simulink library "COR_lib"  (Simulink 7.4)
settings: Solver=FixedStepDiscrete  StartTime=0.0  StopTime=Inf  FixedStep=0.01  RelTol=1e-3
values from neighbouring files (symbols this model uses):
  CORc_fac_CellRDcse_fault = mpt.Parameter    [COR_CAL.m]
  CORc_fac_CellRDcse_warn = mpt.Parameter    [COR_CAL.m]
  CORc_i_ChaEndCur = mpt.Parameter    [COR_CAL.m]
  CORc_i_SOCCrectCurThrld = mpt.Parameter    [COR_CAL.m]
  CORc_pct_DeltSoe_max = mpt.Parameter    [COR_CAL.m]
  CORc_pct_DeltSoe_min = mpt.Parameter    [COR_CAL.m]
  CORc_pct_SOCModValue = mpt.Parameter    [COR_CAL.m]
  CORc_v_CellVoltMax = mpt.Parameter    [COR_CAL.m]
undefined symbols (not defined in the file or in its folder): BATd_iflt_CellCDcse_fault, BATd_pct_CellCVariMax, BATd_pct_CellCVariMin, BATd_v_CellUpperVolt, BATd_v_PackVoltMin, BATm_c_CellChaC_AH, BATm_c_CellDchC_AH, BATm_e_CellSoe, BATm_e_ChaCellSoe, BATm_e_DchCellSoe, BATm_i_PerChaCur, BATm_i_PerDchCur, BATm_i_PulChaCur_limit, BATm_i_PulDchCur_limit, BATm_i_PulDchVolt_limit, BATm_pct_CellCDcseRatio, BATm_pct_CellCycle, BATm_pct_CellSoc, BATm_pct_ChaCellSoc, BATm_pct_DchCellSoc, BATm_pct_SOCofOCVPct, BATm_pct_SohRatio, BATm_r_ChaDcIR, BATm_r_DchDcIR, BATm_v_CellOCV, BATx_pct_CellSocRatio, BATx_pct_PackSoh, BATx_t_CellChaTemp, BATx_t_CellDchTemp, BATx_tm_OfflineTime, BATy_i_CellChaCur, BATy_i_CellDchCur, BATz_v_CellChaVolt, BATz_v_DchCellVolt, BATz_v_DchCellVoltForSoe, BCU_FastCharge_St, BCU_SlowCharge_St, BMS_Const_TickTm_s, BMU_Run_St, FCM_Charging_St, PACK_Const_CellNumOfMdl, PACK_Const_CellNumOfPack, PACK_Const_CycCnt, PACK_Const_MdlNumOfPack, PACK_Const_ParaCellNumOfMdl, PACK_Const_TempSnrNumOfMdl, SCM_Charging_St
libraries: Defined_Functionality x17
(part 2 of 2)

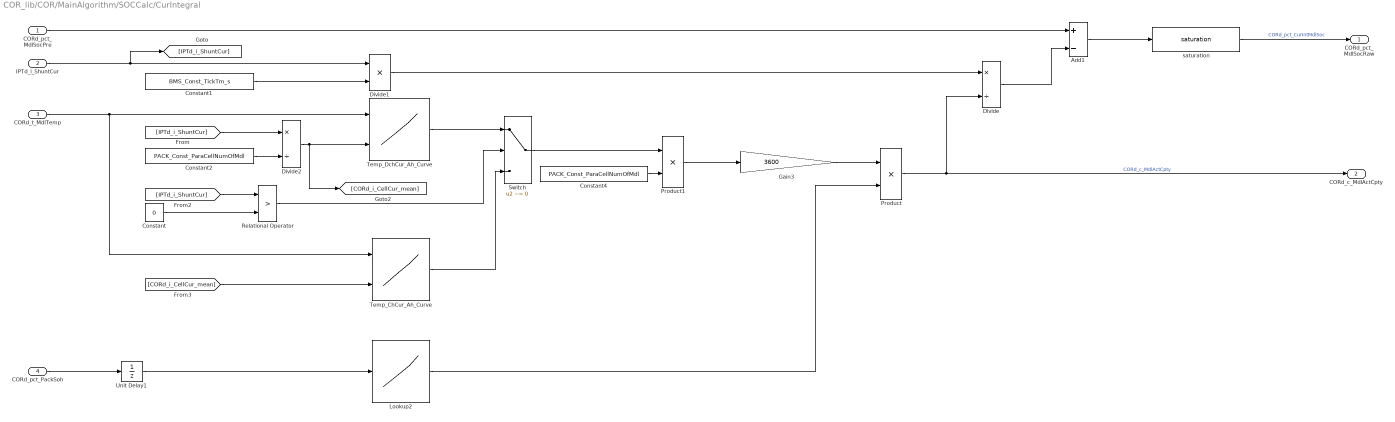
== system COR_lib/COR/MainAlgorithm/SOCCalc/CurIntegral ==
  CORd_pct_MdlSocPre : Inport
  IPTd_i_ShuntCur : Inport  Port=2
  CORd_t_MdlTemp : Inport  Port=3
  CORd_pct_PackSoh : Inport  Port=4  DataType=single  OutDataTypeStr=single
  Add1 : Sum  Inputs=+-
  Constant : Constant  Value=0  OutDataTypeMode=single  OutDataType=fixdt(1, 16)  OutScaling=2^0  OutDataTypeStr=single
  Constant1 : Constant  Value=BMS_Const_TickTm_s  OutDataTypeMode=single  OutDataType=fixdt(1, 16)  OutScaling=2^0  OutDataTypeStr=single
  Constant2 : Constant  Value=PACK_Const_ParaCellNumOfMdl  OutDataTypeMode=single  OutDataType=fixdt(1, 16)  OutScaling=2^0  OutDataTypeStr=single
  Constant4 : Constant  Value=PACK_Const_ParaCellNumOfMdl  OutDataTypeMode=single  OutDataType=fixdt(1, 16)  OutScaling=2^0  OutDataTypeStr=single
  Divide : Product  Inputs=*/
  Divide1 : Product  Inputs=**
  Divide2 : Product  Inputs=*/
  Gain3 : Gain  Gain=3600
  Lookup2 : Lookup  InputValues=BATx_pct_PackSoh  Table=BATm_pct_CellCDcseRatio  LookUpMeth=Interpolation-Use End Values  OutDataType=fixdt(1, 16)  OutScaling=2^0
  Product : Product  OutDataType=fixdt(1, 16)  OutScaling=2^0  RndMeth=Zero
  Product1 : Product  OutDataType=fixdt(1, 16)  OutScaling=2^0  RndMeth=Zero
  Relational Operator : RelationalOperator  Operator=>  LogicOutDataTypeMode=boolean  LogicDataType=fixdt(0, 8)  OutDataTypeStr=boolean
  Switch : Switch  Criteria=u2 ~= 0  OutDataType=fixdt(1, 16)  OutScaling=2^0
  Temp_ChCur_Ah_Curve : Lookup2D  RowIndex=BATx_t_CellChaTemp  ColumnIndex=BATy_i_CellChaCur  Table=BATm_c_CellChaC_AH  LookUpMeth=Interpolation-Use End Values  OutDataType=fixdt(1, 16)  OutScaling=2^0
  Temp_DchCur_Ah_Curve : Lookup2D  RowIndex=BATx_t_CellDchTemp  ColumnIndex=BATy_i_CellDchCur  Table=BATm_c_CellDchC_AH  LookUpMeth=Interpolation-Use End Values  OutDataType=fixdt(1, 16)  OutScaling=2^0
  Unit Delay1 : UnitDelay  SampleTime=-1
  saturation : Defined_Functionality/saturation  SystemSampleTime=-1  upper_limit=1  lower_limit=0
      settings: AttributesFormatString=[UPPER_LIMIT=%<upper_limit>]\n[LOWER_LIMIT=%<lower_limit>]
  CORd_pct_MdlSocRaw : Outport
  CORd_c_MdlActCpty : Outport  Port=2
  wires:
  saturation/1 -> CORd_pct_MdlSocRaw/1  "CORd_pct_CurIntMdlSoc"
  [CORd_i_CellCur_mean] -> Temp_ChCur_Ah_Curve/2
  Divide1/1 -> Divide/1
  Divide/1 -> Add1/2
  Add1/1 -> saturation/1
  IPTd_i_ShuntCur/1 -> [IPTd_i_ShuntCur], Divide1/1
  CORd_t_MdlTemp/1 -> Temp_DchCur_Ah_Curve/1, Temp_ChCur_Ah_Curve/1
  CORd_pct_MdlSocPre/1 -> Add1/1
  [IPTd_i_ShuntCur] -> Relational Operator/1
  Constant/1 -> Relational Operator/2
  Relational Operator/1 -> Switch/2
  Temp_DchCur_Ah_Curve/1 -> Switch/1
  Temp_ChCur_Ah_Curve/1 -> Switch/3
  Switch/1 -> Product1/1
  Constant1/1 -> Divide1/2
  Product/1 -> CORd_c_MdlActCpty/1, Divide/2  "CORd_c_MdlActCpty"
  Lookup2/1 -> Product/2
  CORd_pct_PackSoh/1 -> Unit Delay1/1
  Gain3/1 -> Product/1
  Divide2/1 -> [CORd_i_CellCur_mean], Temp_DchCur_Ah_Curve/2
  [IPTd_i_ShuntCur] -> Divide2/1
  Constant2/1 -> Divide2/2
  Constant4/1 -> Product1/2
  Product1/1 -> Gain3/1
  Unit Delay1/1 -> Lookup2/1

== system COR_lib/COR/MainAlgorithm/SOCCalc/EndSOCCalc ==
  CORd_flg_DchEnd : Inport
  Cord_i_ShuntCur_mean : Inport  Port=2
  CORd_t_MdlTemp : Inport  Port=3
  CORd_v_CellVoltOfMdl_mean : Inport  Port=4
  ChaEndSocCalc : Subsystem
  DchEndSocCalc : Subsystem
  Logical Operator4 : Logic  Operator=NOT  AllPortsSameDT=off  OutDataTypeMode=boolean  LogicDataType=fixdt(0, 8)  OutDataTypeStr=boolean
  Switch : Switch  Criteria=u2 ~= 0  OutDataType=fixdt(1, 16)  OutScaling=2^0
  CORd_pct_EndMdlSoc : Outport
  wires:
  [CORd_t_MdlTemp] -> ChaEndSocCalc/3(CORd_t_MdlTemp)
  [CORd_v_CellVoltOfMdl_mean] -> ChaEndSocCalc/2(CORd_v_CellVoltOfMdl_mean)
  [Cord_i_ShuntCur_mean] -> ChaEndSocCalc/1(Cord_i_ShuntCur_mean)
  Cord_i_ShuntCur_mean/1 -> [Cord_i_ShuntCur_mean], DchEndSocCalc/1(Cord_i_ShuntCur_mean)
  CORd_t_MdlTemp/1 -> DchEndSocCalc/3(CORd_t_MdlTemp), [CORd_t_MdlTemp]
  CORd_v_CellVoltOfMdl_mean/1 -> DchEndSocCalc/2(CORd_v_CellVoltOfMdl_mean), [CORd_v_CellVoltOfMdl_mean]
  DchEndSocCalc/1(CORd_pct_DchEndMdlSoc) -> Switch/1
  Switch/1 -> CORd_pct_EndMdlSoc/1  "CORd_pct_EndMdlSoc"
  [CORd_flg_DchEnd] -> Logical Operator4/1
  Logical Operator4/1 -> ChaEndSocCalc/Enable
  [CORd_flg_DchEnd] -> Switch/2
  CORd_flg_DchEnd/1 -> DchEndSocCalc/Enable, [CORd_flg_DchEnd]
  ChaEndSocCalc/1(CORd_pct_ChEndMdlSoc) -> Switch/3

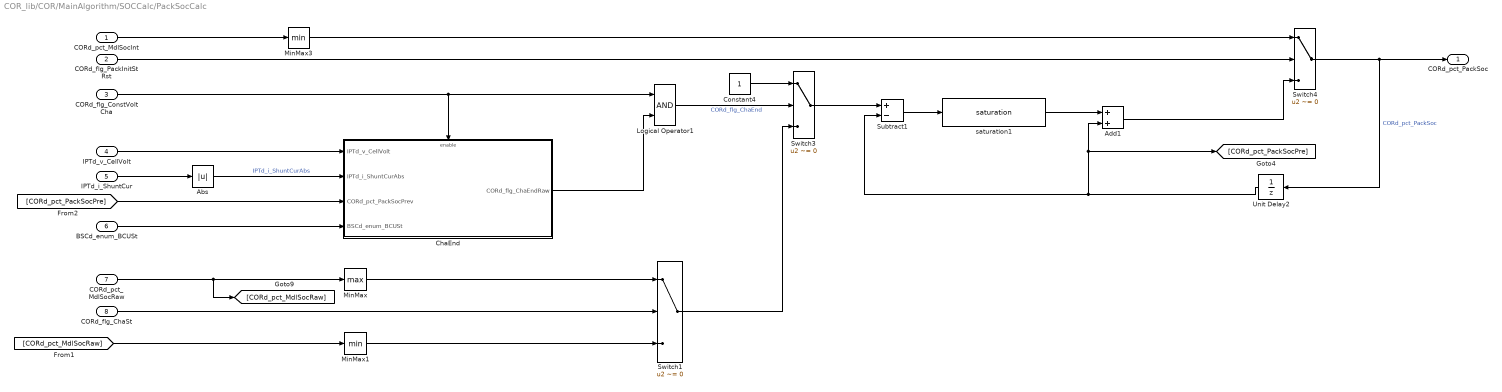
== system COR_lib/COR/MainAlgorithm/SOCCalc/PackSocCalc ==
  CORd_pct_MdlSocInt : Inport
  CORd_flg_PackInitStRst : Inport  Port=2
  CORd_flg_ConstVoltCha : Inport  Port=3
  IPTd_v_CellVolt : Inport  Port=4
  IPTd_i_ShuntCur : Inport  Port=5
  BSCd_enum_BCUSt : Inport  Port=6
  CORd_pct_MdlSocRaw : Inport  Port=7
  CORd_flg_ChaSt : Inport  Port=8
  Abs : Abs  OutDataType=fixdt(1, 16)  OutScaling=2^0
  Add1 : Sum  OutDataType=fixdt(1, 16)  OutScaling=2^-10
  ChaEnd : Subsystem
  Constant4 : Constant  OutDataTypeMode=single  OutDataType=fixdt(1, 16)  OutScaling=2^0  OutDataTypeStr=single
  Logical Operator1 : Logic  AllPortsSameDT=off  OutDataTypeMode=boolean  LogicDataType=fixdt(0, 8)  OutDataTypeStr=boolean
  MinMax : MinMax  Function=max  OutDataType=fixdt(1, 16)  OutScaling=2^0
  MinMax1 : MinMax  OutDataType=fixdt(1, 16)  OutScaling=2^0
  MinMax3 : MinMax  OutDataType=fixdt(1, 16)  OutScaling=2^0
  Subtract1 : Sum  Inputs=+-  OutDataTypeMode=single  OutDataType=fixdt(1, 16)  OutScaling=2^-10  OutDataTypeStr=single
  Switch1 : Switch  Criteria=u2 ~= 0  OutDataType=fixdt(1, 16)  OutScaling=2^0
  Switch3 : Switch  Criteria=u2 ~= 0  OutDataType=fixdt(1, 16)  OutScaling=2^0
  Switch4 : Switch  Criteria=u2 ~= 0  OutDataTypeMode=single  OutDataType=fixdt(1, 16)  OutScaling=2^0  OutDataTypeStr=single
  Unit Delay2 : UnitDelay  SampleTime=-1
  saturation1 : Defined_Functionality/saturation  SystemSampleTime=-1  upper_limit=CORc_pct_DeltSoc_max  lower_limit=CORc_pct_DeltSoc_min
      settings: AttributesFormatString=[UPPER_LIMIT=%<upper_limit>]\n[LOWER_LIMIT=%<lower_limit>]
  CORd_pct_PackSoc : Outport
  wires:
  Switch3/1 -> Subtract1/1
  Unit Delay2/1 -> [CORd_pct_PackSocPre], Add1/2, Subtract1/2
  saturation1/1 -> Add1/1
  MinMax3/1 -> Switch4/1
  Switch4/1 -> CORd_pct_PackSoc/1, Unit Delay2/1  "CORd_pct_PackSoc"
  Subtract1/1 -> saturation1/1
  Add1/1 -> Switch4/3
  CORd_flg_PackInitStRst/1 -> Switch4/2
  CORd_pct_MdlSocInt/1 -> MinMax3/1
  [CORd_pct_MdlSocRaw] -> MinMax1/1
  [CORd_pct_PackSocPre] -> ChaEnd/3(CORd_pct_PackSocPrev)
  Abs/1 -> ChaEnd/2(IPTd_i_ShuntCurAbs)  "IPTd_i_ShuntCurAbs"
  IPTd_i_ShuntCur/1 -> Abs/1
  CORd_flg_ChaSt/1 -> Switch1/2
  Constant4/1 -> Switch3/1
  Logical Operator1/1 -> Switch3/2  "CORd_flg_ChaEnd"
  ChaEnd/1(CORd_flg_ChaEndRaw) -> Logical Operator1/2
  CORd_flg_ConstVoltCha/1 -> ChaEnd/Enable, Logical Operator1/1
  IPTd_v_CellVolt/1 -> ChaEnd/1(IPTd_v_CellVolt)
  Switch1/1 -> Switch3/3
  CORd_pct_MdlSocRaw/1 -> [CORd_pct_MdlSocRaw], MinMax/1
  MinMax1/1 -> Switch1/3
  MinMax/1 -> Switch1/1
  BSCd_enum_BCUSt/1 -> ChaEnd/4(BSCd_enum_BCUSt)

== system COR_lib/COR/MainAlgorithm/SOECalc/EndSoeCalc ==
  CORd_flg_DchEnd : Inport
  CORd_i_ShuntCur_mean : Inport  Port=2
  CORd_v_CellVoltOfMdl_mean : Inport  Port=3
  CORd_t_MdlTemp : Inport  Port=4
  Enable : EnablePort
  ChaEndSoeCal : Subsystem
  DchEndSoeCal : Subsystem
  Logical Operator : Logic  Operator=NOT  AllPortsSameDT=off  OutDataTypeMode=boolean  LogicDataType=fixdt(0, 8)  OutDataTypeStr=boolean
  Switch : Switch  Criteria=u2 ~= 0  OutDataType=fixdt(1, 16)  OutScaling=2^0
  CORd_e_PackSoeRaw2 : Outport
  wires:
  [CORd_t_MdlTemp] -> ChaEndSoeCal/3(CORd_t_MdlTemp)
  [CORd_v_CellVoltOfMdl_mean] -> ChaEndSoeCal/2(CORd_v_CellVoltOfMdl_mean)
  CORd_t_MdlTemp/1 -> [CORd_t_MdlTemp], DchEndSoeCal/3(CORd_t_MdlTemp)
  CORd_v_CellVoltOfMdl_mean/1 -> [CORd_v_CellVoltOfMdl_mean], DchEndSoeCal/2(CORd_v_CellVoltOfMdl_mean)
  [CORd_i_ShuntCur_mean] -> ChaEndSoeCal/1(CORd_i_ShuntCur_mean)
  Switch/1 -> CORd_e_PackSoeRaw2/1  "CORd_e_PackSoeRaw2"
  DchEndSoeCal/1(CORd_e_DchEndCellSoc) -> Switch/1
  ChaEndSoeCal/1(CORd_e_ChaEndCellSoc) -> Switch/3
  CORd_flg_DchEnd/1 -> DchEndSoeCal/Enable, [CORd_flg_DchEnd]
  [CORd_flg_DchEnd] -> Switch/2
  [CORd_flg_DchEnd] -> Logical Operator/1
  Logical Operator/1 -> ChaEndSoeCal/Enable
  CORd_i_ShuntCur_mean/1 -> DchEndSoeCal/1(CORd_i_ShuntCur_mean), [CORd_i_ShuntCur_mean]

== system COR_lib/COR/MainAlgorithm/SOECalc/PackDC-IRCalc ==
  CORd_t_MdlTemp : Inport
  CORd_pct_MdlSoc : Inport  Port=2
  IPTd_i_ShuntCur : Inport  Port=3
  Constant : Constant  OutDataTypeMode=single  OutDataType=fixdt(1, 16)  OutScaling=2^0  OutDataTypeStr=single
  Constant1 : Constant  Value=1000  OutDataTypeMode=single  OutDataType=fixdt(1, 16)  OutScaling=2^0  OutDataTypeStr=single
  Constant2 : Constant  Value=-1  OutDataTypeMode=single  OutDataType=fixdt(1, 16)  OutScaling=2^0  OutDataTypeStr=single
  Constant3 : Constant  Value=0  OutDataTypeMode=single  OutDataType=fixdt(1, 16)  OutScaling=2^0  OutDataTypeStr=single
  Constant4 : Constant  Value=PACK_Const_ParaCellNumOfMdl  OutDataTypeMode=single  OutDataType=fixdt(1, 16)  OutScaling=2^0  OutDataTypeStr=single
  Constant5 : Constant  Value=PACK_Const_CellNumOfMdl  OutDataTypeMode=single  OutDataType=fixdt(1, 16)  OutScaling=2^0  OutDataTypeStr=single
  Divide : Product  Inputs=*/  OutDataType=fixdt(1, 16)  OutScaling=2^-10
  Divide1 : Product  Inputs=*/  OutDataType=fixdt(1, 16)  OutScaling=2^-10
  Product : Product  OutDataType=fixdt(1, 16)  OutScaling=2^0  RndMeth=Zero
  Relational Operator : RelationalOperator  Operator=>  LogicOutDataTypeMode=boolean  LogicDataType=fixdt(0, 8)  OutDataTypeStr=boolean
  Relational Operator1 : RelationalOperator  Operator=<  LogicOutDataTypeMode=boolean  LogicDataType=fixdt(0, 8)  OutDataTypeStr=boolean
  Sum of Elements3 : Sum  Inputs=+  CollapseDim=2  OutDataType=fixdt(1, 16)  OutScaling=2^-10
  Switch : Switch  Criteria=u2 ~= 0  OutDataType=fixdt(1, 16)  OutScaling=2^0
  Switch1 : Switch  Criteria=u2 ~= 0  OutDataType=fixdt(1, 16)  OutScaling=2^0
  T_SOC_ChaDcIR : Lookup2D  RowIndex=BATx_t_CellDchTemp  ColumnIndex=BATy_pct_CellSoc  Table=BATm_r_ChaDcIR  LookUpMeth=Interpolation-Use End Values  OutDataType=fixdt(1, 16)  OutScaling=2^0
  T_SOC_DchDcIR : Lookup2D  RowIndex=BATx_t_CellDchTemp  ColumnIndex=BATy_pct_CellSoc  Table=BATm_r_DchDcIR  LookUpMeth=Interpolation-Use End Values  OutDataTypeMode=single  OutDataType=fixdt(1, 16)  OutScaling=2^0  OutDataTypeStr=single
  CORd_r_CellDCIR : Outport  OutDataType=fixdt(1, 16)  OutScaling=2^0
  CORd_r_PackDCIR : Outport  Port=2  OutDataType=fixdt(1, 16)  OutScaling=2^0
  wires:
  Product/1 -> Sum of Elements3/1
  Divide/1 -> CORd_r_PackDCIR/1  "CORd_r_PackDCIR"
  CORd_t_MdlTemp/1 -> T_SOC_DchDcIR/1, [CORd_t_MdlTemp]
  CORd_pct_MdlSoc/1 -> [CORd_pct_MdlSoc], T_SOC_DchDcIR/2
  IPTd_i_ShuntCur/1 -> Relational Operator/1, Relational Operator1/1
  Constant/1 -> Relational Operator/2
  Relational Operator/1 -> Switch/2
  Switch/1 -> Product/1, CORd_r_CellDCIR/1  "CORd_r_CellDCIR"
  [CORd_pct_MdlSoc] -> T_SOC_ChaDcIR/2
  T_SOC_DchDcIR/1 -> Switch/1
  Constant1/1 -> Divide/2
  [CORd_t_MdlTemp] -> T_SOC_ChaDcIR/1
  T_SOC_ChaDcIR/1 -> Switch1/1
  Constant2/1 -> Relational Operator1/2
  Relational Operator1/1 -> Switch1/2
  Constant3/1 -> Switch1/3
  Switch1/1 -> Switch/3
  Sum of Elements3/1 -> Divide1/1
  Constant4/1 -> Divide1/2
  Divide1/1 -> Divide/1
  Constant5/1 -> Product/2

== system COR_lib/COR/MainAlgorithm/SOECalc/PowInt ==
  note: Note:Not include the energy consumed by the terminals.
  CORd_r_PackDCIR : Inport
  CORd_e_PackSoePre : Inport  Port=2
  CORd_v_CellVoltOfMdl_mean : Inport  Port=3
  IPTd_i_ShuntCur : Inport  Port=4
  Add1 : Sum  Inputs=+-
  Add2 : Sum
  Constant : Constant  Value=3600  OutDataTypeMode=single  OutDataType=fixdt(1, 16)  OutScaling=2^0  OutDataTypeStr=single
  Constant2 : Constant  Value=BMS_Const_TickTm_s  OutDataTypeMode=single  OutDataType=fixdt(1, 16)  OutScaling=2^0  OutDataTypeStr=single
  Constant3 : Constant  Value=3600  OutDataTypeMode=single  OutDataType=fixdt(1, 16)  OutScaling=2^0  OutDataTypeStr=single
  Constant4 : Constant  Value=PACK_Const_CellNumOfMdl  OutDataTypeMode=single  OutDataType=fixdt(1, 16)  OutScaling=2^0  OutDataTypeStr=single
  Divide : Product  Inputs=*/  OutDataType=fixdt(1, 16)  OutScaling=2^-10  OutDataTypeStr=Inherit: Inherit via back propagation
  Divide{1,3..7} (6 alike) : Product  Inputs=**
  Sum of Elements : Sum  Inputs=+  OutDataType=fixdt(1, 16)  OutScaling=2^-10
  CORd_e_PackSoeRaw1 : Outport
  wires:
  Divide5/1 -> Add1/2
  Constant4/1 -> Divide7/2
  Constant3/1 -> Divide6/2
  IPTd_i_ShuntCur/1 -> Divide1/2, Divide4/1, Divide4/2
  Add1/1 -> Divide/1
  CORd_v_CellVoltOfMdl_mean/1 -> Sum of Elements/1
  Divide1/1 -> Add2/1
  CORd_r_PackDCIR/1 -> Divide3/2
  Constant/1 -> Divide/2
  Sum of Elements/1 -> Divide7/1
  Divide4/1 -> Divide3/1
  Divide3/1 -> Add2/2
  Constant2/1 -> Divide5/2
  Divide7/1 -> Divide1/1
  CORd_e_PackSoePre/1 -> Divide6/1
  Divide6/1 -> Add1/1
  Add2/1 -> Divide5/1
  Divide/1 -> CORd_e_PackSoeRaw1/1  "CORd_e_PackSoeRaw1"

== system COR_lib/COR/MainAlgorithm/SOHCalc/SohBaseCycle ==
  CORd_num_RemdCycInt : Inport
  IPTd_i_ShuntCur : Inport  Port=2
  CORd_c_MdlActCpty : Inport  Port=3
  CORd_t_MdlTemp : Inport  Port=4
  Abs : Abs  OutDataType=fixdt(1, 16)  OutScaling=2^0
  Add1 : Sum  Inputs=+-
  Constant : Constant  Value=2  OutDataTypeMode=uint8  OutDataType=fixdt(1, 16)  OutScaling=2^0  OutDataTypeStr=uint8
  Constant1 : Constant  Value=BMS_Const_TickTm_s  OutDataTypeMode=single  OutDataType=fixdt(1, 16)  OutScaling=2^0  OutDataTypeStr=single
  Constant5 : Constant  Value=PACK_Const_CycCnt  OutDataTypeMode=single  OutDataType=fixdt(1, 16)  OutScaling=2^0  OutDataTypeStr=single
  Constant6 : Constant  Value=PACK_Const_MdlNumOfPack  OutDataTypeMode=uint8  OutDataType=fixdt(1, 16)  OutScaling=2^0  OutDataTypeStr=uint8
  Divide : Product  Inputs=*/
  Divide1 : Product  Inputs=**
  Divide2 : Product  Inputs=*/
  Divide3 : Product  Inputs=*/  OutDataType=fixdt(1, 16)  OutScaling=2^-10
  Divide4 : Product  Inputs=*/  OutDataTypeStr=Inherit: Inherit via back propagation
  Divide5 : Product  Inputs=**
  Sum of Elements : Sum  Inputs=+  OutDataType=fixdt(1, 16)  OutScaling=2^-10
  Temp_DchCur_SohRatio : Lookup2D  RowIndex=BATx_t_CellDchTemp  ColumnIndex=BATy_i_CellDchCur  Table=BATm_pct_SohRatio  LookUpMeth=Interpolation-Use End Values  OutDataType=fixdt(1, 16)  OutScaling=2^0
  integrator : Defined_Functionality/integrator  SystemSampleTime=-1  Initial_Value=0
  CORd_num_RemdCycle1 : Outport
  CORd_pct_PackSoh1 : Outport  Port=2
  wires:
  Divide1/1 -> integrator/1
  integrator/1 -> Divide/1
  Divide2/1 -> Divide5/1
  Divide/1 -> Divide2/1
  Constant/1 -> Divide2/2
  Abs/1 -> Divide1/2, [CORd_i_ShuntCurAbs]
  Constant1/1 -> Divide1/1
  IPTd_i_ShuntCur/1 -> Abs/1
  Constant6/1 -> Divide3/2
  Divide3/1 -> Add1/2
  Sum of Elements/1 -> Divide3/1
  Constant5/1 -> Divide4/2
  Divide4/1 -> CORd_pct_PackSoh1/1
  Add1/1 -> Divide4/1, CORd_num_RemdCycle1/1
  CORd_num_RemdCycInt/1 -> Add1/1
  CORd_c_MdlActCpty/1 -> Divide/2
  Divide5/1 -> Sum of Elements/1
  Temp_DchCur_SohRatio/1 -> Divide5/2
  [CORd_i_ShuntCurAbs] -> Temp_DchCur_SohRatio/2
  CORd_t_MdlTemp/1 -> Temp_DchCur_SohRatio/1

== system COR_lib/COR/MainAlgorithm/SOHCalc/SohUpdate ==
  CORd_flg_ChaSt : Inport
  CORd_pct_MdlSoc : Inport  Port=2
  CORd_pct_PackSohPre : Inport  Port=3
  IPTd_i_ShuntCur : Inport  Port=4
  CORd_t_MdlTemp : Inport  Port=5
  CORd_flg_ConstVoltCha : Inport  Port=6
  ChaCapacityCal : Subsystem
  ChaIntSoc : Subsystem
  ChargingSt : Subsystem
  ChargingSt1 : Subsystem
  Data Store Memory : DataStoreMemory  DataStoreName=CORd_c_ChaC  ReadBeforeWriteMsg=warning  WriteAfterWriteMsg=warning  WriteAfterReadMsg=warning  OutDataType=fixdt(1, 16)  OutScaling=2^0
  Data Store Write1 : DataStoreWrite  DataStoreName=CORd_c_ChaC  SampleTime=-1
  Soh2Update : Subsystem
  CORd_pct_PackSoh2 : Outport  OutDataType=fixdt(1, 16)  OutScaling=2^0
  CORd_num_RemdCycle2 : Outport  Port=2  OutDataType=fixdt(1, 16)  OutScaling=2^0
  CORd_iflt_CellCDcse_fault : Outport  Port=3  OutDataType=fixdt(1, 16)  OutScaling=2^0
  wires:
  ChargingSt1/1(ChargingSt) -> ChaIntSoc/Enable
  [CORd_pct_MdlSoc] -> Soh2Update/2(CORd_pct_MdlSoc)
  [CORd_flg_ChaSt] -> ChaCapacityCal/Enable
  ChargingSt/1(ChargingSt) -> Soh2Update/Enable
  Soh2Update/2(CORd_iflt_CellCDcse_fault) -> CORd_iflt_CellCDcse_fault/1
  CORd_flg_ConstVoltCha/1 -> ChaCapacityCal/3(CORd_flg_ConstVoltCha)
  CORd_t_MdlTemp/1 -> ChaCapacityCal/2(CORd_t_MdlTemp)
  IPTd_i_ShuntCur/1 -> ChaCapacityCal/1(IPTd_i_ShuntCur)
  CORd_pct_PackSohPre/1 -> Soh2Update/6(CORd_pct_PackSohPre)
  Soh2Update/1(CORd_pct_PackSoh2) -> CORd_pct_PackSoh2/1
  ChaCapacityCal/3(CORd_i_ChaCurAvrage) -> Soh2Update/5(CORd_i_ChaCurAvrage)
  ChaCapacityCal/2(CORd_t_ChaTempAvrage) -> Soh2Update/4(CORd_t_ChaTempAvrage)
  ChaCapacityCal/1(CORd_c_ChaCRaw) -> Data Store Write1/1, Soh2Update/3(CORd_c_ChaCRaw)
  CORd_flg_ChaSt/1 -> ChargingSt1/1(CORd_flg_ChaSt), ChargingSt/1(CORd_flg_ChaSt), [CORd_flg_ChaSt]
  ChaIntSoc/1(CORd_pct_ChaInSoc) -> Soh2Update/1(CORd_pct_ChaIntSoc)
  CORd_pct_MdlSoc/1 -> ChaIntSoc/1(CORd_pct_MdlSoc), [CORd_pct_MdlSoc]
  Soh2Update/3(CORd_num_RemdCycle2) -> CORd_num_RemdCycle2/1

== system COR_lib/COR/MainAlgorithm/CellOhmRObs/CellOhmRCal/Subsystem ==
  CORd_i_CurSnrDelta : Inport
  CORd_v_CellVoltOfMdl_Mean : Inport  Port=2
  CORd_t_CellTemp : Inport  Port=3
  CORd_pct_CellSoc : Inport  Port=4
  Enable : EnablePort
  Add1 : Sum  Inputs=-+  OutDataType=fixdt(1, 16)  OutScaling=2^-10
  Add2 : Sum  Inputs=+-  OutDataType=fixdt(1, 16)  OutScaling=2^-10
  Bus Creator : BusCreator  Inputs=2
  Bus Creator1 : BusCreator  Inputs=2
  Bus Creator2 : BusCreator  Inputs=2
  Demux : Demux  Outputs=2
  Divide : Product  Inputs=*/  OutDataType=fixdt(1, 16)  OutScaling=2^-10
  T_SOC_OCV : Lookup2D  RowIndex=BATx_t_CellTemp  ColumnIndex=BATy_pct_CellSocForOCV  Table=BATm_v_CellOCV  LookUpMeth=Interpolation-Use End Values  OutDataType=fixdt(1, 16)  OutScaling=2^0
  Unit Delay1 : UnitDelay  SampleTime=-1
  Unit Delay2 : UnitDelay  SampleTime=-1
  Unit Delay3 : UnitDelay  SampleTime=-1
  CORd_r_CellOhmR : Outport
  wires:
  CORd_v_CellVoltOfMdl_Mean/1 -> Unit Delay3/1, Bus Creator/1
  CORd_t_CellTemp/1 -> Unit Delay1/1, Bus Creator1/1
  Unit Delay1/1 -> Bus Creator1/2
  Bus Creator1/1 -> T_SOC_OCV/1
  CORd_pct_CellSoc/1 -> Bus Creator2/1, Unit Delay2/1
  Unit Delay2/1 -> Bus Creator2/2
  Bus Creator2/1 -> T_SOC_OCV/2
  Unit Delay3/1 -> Bus Creator/2
  Bus Creator/1 -> Add1/1
  T_SOC_OCV/1 -> Add1/2
  Add1/1 -> Demux/1
  Demux/1 -> Add2/1
  Add2/1 -> Divide/2
  Demux/2 -> Add2/2
  CORd_i_CurSnrDelta/1 -> Divide/1
  Divide/1 -> CORd_r_CellOhmR/1  "CORd_r_CellOhmR"

== system COR_lib/COR/MainAlgorithm/SOCCalc/EndSOCCalc/ChaEndSocCalc ==
  Cord_i_ShuntCur_mean : Inport
  CORd_v_CellVoltOfMdl_mean : Inport  Port=2
  CORd_t_MdlTemp : Inport  Port=3
  Enable : EnablePort
  ChCur_Volt_Temp_Cofficient : Lookup_n-D  NumberOfTableDimensions=3  BreakpointsForDimension1=BATy_i_CellChaCur  BreakpointsForDimension2=BATz_v_CellChaVolt  BreakpointsForDimension3=BATx_t_CellChaTemp  Table=BATm_pct_ChaCellSoc  TableDataTypeStr=Inherit: Inherit from 'Table data'  OutDataTypeStr=single  InputSameDT=on
  Constant4 : Constant  Value=PACK_Const_ParaCellNumOfMdl  OutDataType=fixdt(1, 16)  OutScaling=2^0
  Divide : Product  Inputs=*/  OutDataType=fixdt(1, 16)  OutScaling=2^-10  OutDataTypeStr=Inherit: Inherit via back propagation
  saturation : Defined_Functionality/saturation  SystemSampleTime=-1  upper_limit=1  lower_limit=0
      settings: AttributesFormatString=[UPPER_LIMIT=%<upper_limit>]\n[LOWER_LIMIT=%<lower_limit>]
  CORd_pct_ChEndMdlSoc : Outport
  wires:
  saturation/1 -> CORd_pct_ChEndMdlSoc/1  "CORd_pct_ChEndMdlSoc"
  ChCur_Volt_Temp_Cofficient/1 -> saturation/1
  Cord_i_ShuntCur_mean/1 -> Divide/1
  CORd_v_CellVoltOfMdl_mean/1 -> ChCur_Volt_Temp_Cofficient/2
  CORd_t_MdlTemp/1 -> ChCur_Volt_Temp_Cofficient/3
  Constant4/1 -> Divide/2
  Divide/1 -> ChCur_Volt_Temp_Cofficient/1

== system COR_lib/COR/MainAlgorithm/SOCCalc/EndSOCCalc/DchEndSocCalc ==
  Cord_i_ShuntCur_mean : Inport
  CORd_v_CellVoltOfMdl_mean : Inport  Port=2
  CORd_t_MdlTemp : Inport  Port=3
  Enable : EnablePort
  Constant4 : Constant  Value=PACK_Const_ParaCellNumOfMdl  OutDataType=fixdt(1, 16)  OutScaling=2^0
  DchCur_Volt_Temp_Cofficient : Lookup_n-D  NumberOfTableDimensions=3  BreakpointsForDimension1=BATy_i_CellDchCur  BreakpointsForDimension2=BATz_v_DchCellVolt  BreakpointsForDimension3=BATx_t_CellDchTemp  Table=BATm_pct_DchCellSoc  TableDataTypeStr=Inherit: Inherit from 'Table data'  OutDataTypeStr=single  InputSameDT=on
  Divide : Product  Inputs=*/  OutDataType=fixdt(1, 16)  OutScaling=2^-10  OutDataTypeStr=Inherit: Inherit via back propagation
  saturation : Defined_Functionality/saturation  SystemSampleTime=-1  upper_limit=1  lower_limit=0
      settings: AttributesFormatString=[UPPER_LIMIT=%<upper_limit>]\n[LOWER_LIMIT=%<lower_limit>]
  CORd_pct_DchEndMdlSoc : Outport
  wires:
  saturation/1 -> CORd_pct_DchEndMdlSoc/1  "CORd_pct_DchEndCellSoc"
  Cord_i_ShuntCur_mean/1 -> Divide/1
  CORd_v_CellVoltOfMdl_mean/1 -> DchCur_Volt_Temp_Cofficient/2
  CORd_t_MdlTemp/1 -> DchCur_Volt_Temp_Cofficient/3
  DchCur_Volt_Temp_Cofficient/1 -> saturation/1
  Constant4/1 -> Divide/2
  Divide/1 -> DchCur_Volt_Temp_Cofficient/1

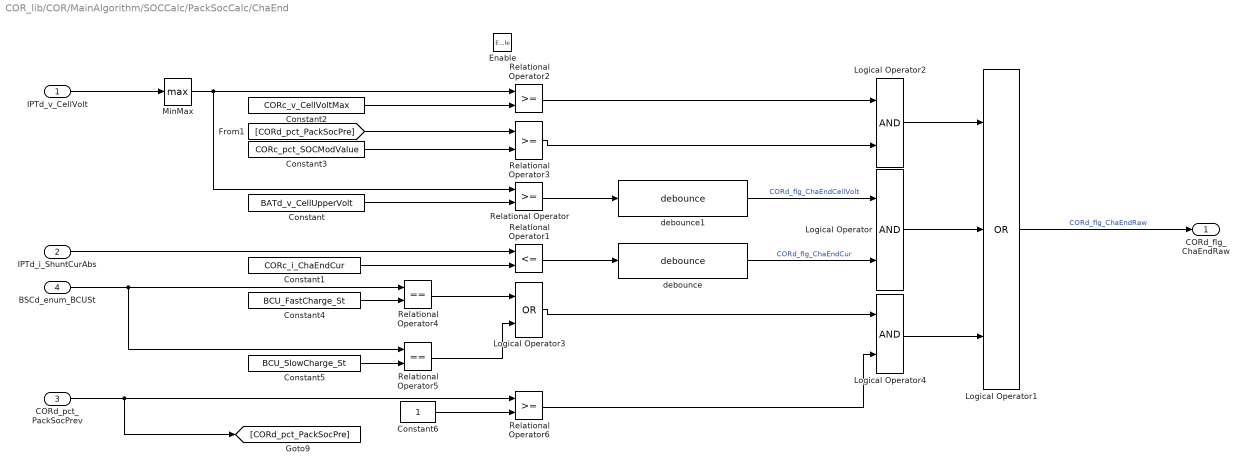
== system COR_lib/COR/MainAlgorithm/SOCCalc/PackSocCalc/ChaEnd ==
  IPTd_v_CellVolt : Inport
  IPTd_i_ShuntCurAbs : Inport  Port=2
  CORd_pct_PackSocPrev : Inport  Port=3
  BSCd_enum_BCUSt : Inport  Port=4
  Enable : EnablePort
  Constant : Constant  Value=BATd_v_CellUpperVolt  OutDataTypeMode=single  OutDataType=fixdt(1, 16)  OutScaling=2^0  OutDataTypeStr=single
  Constant1 : Constant  Value=CORc_i_ChaEndCur  OutDataTypeMode=single  OutDataType=fixdt(1, 16)  OutScaling=2^0  OutDataTypeStr=single
  Constant2 : Constant  Value=CORc_v_CellVoltMax  OutDataTypeMode=single  OutDataType=fixdt(1, 16)  OutScaling=2^0  OutDataTypeStr=single
  Constant3 : Constant  Value=CORc_pct_SOCModValue  OutDataTypeMode=single  OutDataType=fixdt(1, 16)  OutScaling=2^0  OutDataTypeStr=single
  Constant4 : Constant  Value=BCU_FastCharge_St  OutDataTypeMode=single  OutDataType=fixdt(1, 16)  OutScaling=2^0  OutDataTypeStr=single
  Constant5 : Constant  Value=BCU_SlowCharge_St  OutDataTypeMode=single  OutDataType=fixdt(1, 16)  OutScaling=2^0  OutDataTypeStr=single
  Constant6 : Constant  OutDataTypeMode=single  OutDataType=fixdt(1, 16)  OutScaling=2^0  OutDataTypeStr=single
  Logical Operator : Logic  AllPortsSameDT=off  OutDataTypeMode=boolean  LogicDataType=fixdt(0, 8)  OutDataTypeStr=boolean
  Logical Operator1 : Logic  Operator=OR  Inputs=3  AllPortsSameDT=off  OutDataTypeMode=boolean  LogicDataType=fixdt(0, 8)  OutDataTypeStr=boolean
  Logical Operator2 : Logic  AllPortsSameDT=off  OutDataTypeMode=boolean  LogicDataType=fixdt(0, 8)  OutDataTypeStr=boolean
  Logical Operator3 : Logic  Operator=OR  AllPortsSameDT=off  OutDataTypeMode=boolean  LogicDataType=fixdt(0, 8)  OutDataTypeStr=boolean
  Logical Operator4 : Logic  AllPortsSameDT=off  OutDataTypeMode=boolean  LogicDataType=fixdt(0, 8)  OutDataTypeStr=boolean
  MinMax : MinMax  Function=max  OutDataType=fixdt(1, 16)  OutScaling=2^0  OutDataTypeStr=Inherit: Inherit via back propagation
  Relational Operator{,2..3,6} (4 alike) : RelationalOperator  LogicOutDataTypeMode=boolean  LogicDataType=fixdt(0, 8)  OutDataTypeStr=boolean
  Relational Operator1 : RelationalOperator  Operator=<=  LogicOutDataTypeMode=boolean  LogicDataType=fixdt(0, 8)  OutDataTypeStr=boolean
  Relational Operator4 : RelationalOperator  Operator===  LogicOutDataTypeMode=boolean  LogicDataType=fixdt(0, 8)  OutDataTypeStr=boolean
  Relational Operator5 : RelationalOperator  Operator===  LogicOutDataTypeMode=boolean  LogicDataType=fixdt(0, 8)  OutDataTypeStr=boolean
  debounce : Defined_Functionality/debounce  SystemSampleTime=-1  debounce_time=CORc_tm_CurAbsUnder
      settings: AttributesFormatString=[DEBOUNCE_TIME=%<debounce_time>]
  debounce1 : Defined_Functionality/debounce  SystemSampleTime=-1  debounce_time=CORc_tm_CellVoltOver
      settings: AttributesFormatString=[DEBOUNCE_TIME=%<debounce_time>]
  CORd_flg_ChaEndRaw : Outport  OutDataType=fixdt(1, 16)  OutScaling=2^0
  wires:
  MinMax/1 -> Relational Operator/1, Relational Operator2/1
  Relational Operator3/1 -> Logical Operator2/2
  Constant3/1 -> Relational Operator3/2
  Logical Operator2/1 -> Logical Operator1/1
  Relational Operator2/1 -> Logical Operator2/1
  Constant2/1 -> Relational Operator2/2
  Logical Operator1/1 -> CORd_flg_ChaEndRaw/1  "CORd_flg_ChaEndRaw"
  Logical Operator/1 -> Logical Operator1/2
  debounce/1 -> Logical Operator/2  "CORd_flg_ChaEndCur"
  debounce1/1 -> Logical Operator/1  "CORd_flg_ChaEndCellVolt"
  IPTd_v_CellVolt/1 -> MinMax/1
  Constant/1 -> Relational Operator/2
  IPTd_i_ShuntCurAbs/1 -> Relational Operator1/1
  Constant1/1 -> Relational Operator1/2
  Relational Operator/1 -> debounce1/1
  Relational Operator1/1 -> debounce/1
  BSCd_enum_BCUSt/1 -> Relational Operator4/1, Relational Operator5/1
  Relational Operator4/1 -> Logical Operator3/1
  Constant4/1 -> Relational Operator4/2
  Constant5/1 -> Relational Operator5/2
  Relational Operator5/1 -> Logical Operator3/2
  Logical Operator3/1 -> Logical Operator4/1
  Logical Operator4/1 -> Logical Operator1/3
  CORd_pct_PackSocPrev/1 -> [CORd_pct_PackSocPre], Relational Operator6/1
  [CORd_pct_PackSocPre] -> Relational Operator3/1
  Relational Operator6/1 -> Logical Operator4/2
  Constant6/1 -> Relational Operator6/2

== system COR_lib/COR/MainAlgorithm/SOECalc/EndSoeCalc/ChaEndSoeCal ==
  CORd_i_ShuntCur_mean : Inport
  CORd_v_CellVoltOfMdl_mean : Inport  Port=2
  CORd_t_MdlTemp : Inport  Port=3
  Enable : EnablePort
  ChaCurVSVoltTable2 : Lookup_n-D  NumberOfTableDimensions=3  BreakpointsForDimension1=BATy_i_CellChaCur  BreakpointsForDimension2=BATz_v_CellChaVolt  BreakpointsForDimension3=BATx_t_CellChaTemp  Table=BATm_e_ChaCellSoe  TableDataTypeStr=Inherit: Inherit from 'Table data'  OutDataTypeStr=single  InputSameDT=on
  Constant1 : Constant  Value=PACK_Const_ParaCellNumOfMdl  OutDataTypeMode=single  OutDataType=fixdt(1, 16)  OutScaling=2^0  OutDataTypeStr=single
  Constant2 : Constant  Value=PACK_Const_ParaCellNumOfMdl  OutDataTypeMode=uint8  OutDataType=fixdt(1, 16)  OutScaling=2^0  OutDataTypeStr=uint8
  Constant3 : Constant  Value=PACK_Const_CellNumOfPack  OutDataTypeMode=uint8  OutDataType=fixdt(1, 16)  OutScaling=2^0  OutDataTypeStr=uint8
  Divide : Product  Inputs=*/  OutDataType=fixdt(1, 16)  OutScaling=2^-10
  MinMax : MinMax  OutDataType=fixdt(1, 16)  OutScaling=2^0
  Product1 : Product  OutDataType=fixdt(1, 16)  OutScaling=2^0  RndMeth=Zero
  Product2 : Product  OutDataType=fixdt(1, 16)  OutScaling=2^0  RndMeth=Zero
  CORd_e_ChaEndCellSoc : Outport
  wires:
  Divide/1 -> ChaCurVSVoltTable2/1
  CORd_i_ShuntCur_mean/1 -> Divide/1
  Constant1/1 -> Divide/2
  CORd_v_CellVoltOfMdl_mean/1 -> ChaCurVSVoltTable2/2
  CORd_t_MdlTemp/1 -> ChaCurVSVoltTable2/3
  MinMax/1 -> Product2/1
  ChaCurVSVoltTable2/1 -> MinMax/1
  Product2/1 -> CORd_e_ChaEndCellSoc/1
  Constant3/1 -> Product1/1
  Constant2/1 -> Product1/2
  Product1/1 -> Product2/2

== system COR_lib/COR/MainAlgorithm/SOECalc/EndSoeCalc/DchEndSoeCal ==
  CORd_i_ShuntCur_mean : Inport
  CORd_v_CellVoltOfMdl_mean : Inport  Port=2
  CORd_t_MdlTemp : Inport  Port=3
  Enable : EnablePort
  ChaCur_Volt_Temp_Soe : Lookup_n-D  NumberOfTableDimensions=3  BreakpointsForDimension1=BATy_i_CellDchCur  BreakpointsForDimension2=BATz_v_DchCellVoltForSoe  BreakpointsForDimension3=BATx_t_CellDchTemp  Table=BATm_e_DchCellSoe  TableDataTypeStr=Inherit: Inherit from 'Table data'  OutDataTypeStr=single  InputSameDT=on
  Constant1 : Constant  Value=PACK_Const_ParaCellNumOfMdl  OutDataTypeMode=single  OutDataType=fixdt(1, 16)  OutScaling=2^0  OutDataTypeStr=single
  Constant2 : Constant  Value=PACK_Const_ParaCellNumOfMdl  OutDataTypeMode=uint8  OutDataType=fixdt(1, 16)  OutScaling=2^0  OutDataTypeStr=uint8
  Constant4 : Constant  Value=PACK_Const_CellNumOfPack  OutDataTypeMode=uint8  OutDataType=fixdt(1, 16)  OutScaling=2^0  OutDataTypeStr=uint8
  Divide : Product  Inputs=*/  OutDataType=fixdt(1, 16)  OutScaling=2^-10
  MinMax : MinMax  OutDataType=fixdt(1, 16)  OutScaling=2^0
  Product1 : Product  OutDataType=fixdt(1, 16)  OutScaling=2^0  RndMeth=Zero
  Product2 : Product  OutDataType=fixdt(1, 16)  OutScaling=2^0  RndMeth=Zero
  CORd_e_DchEndCellSoc : Outport
  wires:
  Divide/1 -> ChaCur_Volt_Temp_Soe/1
  CORd_i_ShuntCur_mean/1 -> Divide/1
  Constant1/1 -> Divide/2
  CORd_t_MdlTemp/1 -> ChaCur_Volt_Temp_Soe/3
  CORd_v_CellVoltOfMdl_mean/1 -> ChaCur_Volt_Temp_Soe/2
  Product2/1 -> CORd_e_DchEndCellSoc/1
  ChaCur_Volt_Temp_Soe/1 -> MinMax/1
  MinMax/1 -> Product2/1
  Constant4/1 -> Product1/1
  Constant2/1 -> Product1/2
  Product1/1 -> Product2/2

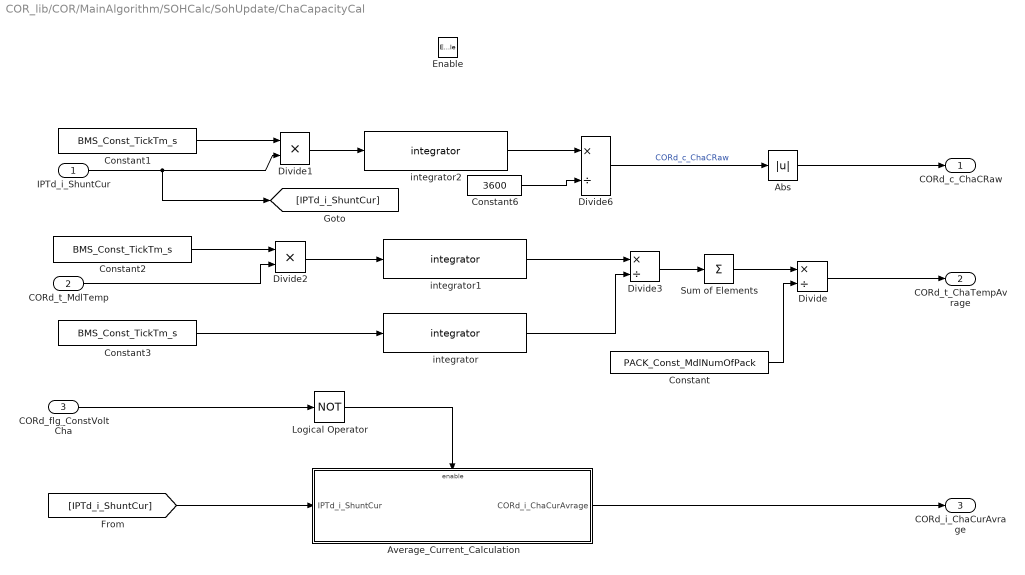
== system COR_lib/COR/MainAlgorithm/SOHCalc/SohUpdate/ChaCapacityCal ==
  IPTd_i_ShuntCur : Inport
  CORd_t_MdlTemp : Inport  Port=2
  CORd_flg_ConstVoltCha : Inport  Port=3
  Enable : EnablePort
  Abs : Abs  OutDataType=fixdt(1, 16)  OutScaling=2^0
  Average_Current_Calculation : Subsystem
  Constant : Constant  Value=PACK_Const_MdlNumOfPack  OutDataTypeMode=single  OutDataType=fixdt(1, 16)  OutScaling=2^0  OutDataTypeStr=single
  Constant1 : Constant  Value=BMS_Const_TickTm_s  OutDataTypeMode=single  OutDataType=fixdt(1, 16)  OutScaling=2^0  OutDataTypeStr=single
  Constant2 : Constant  Value=BMS_Const_TickTm_s  OutDataTypeMode=single  OutDataType=fixdt(1, 16)  OutScaling=2^0  OutDataTypeStr=single
  Constant3 : Constant  Value=BMS_Const_TickTm_s  OutDataTypeMode=single  OutDataType=fixdt(1, 16)  OutScaling=2^0  OutDataTypeStr=single
  Constant6 : Constant  Value=3600  OutDataTypeMode=single  OutDataType=fixdt(1, 16)  OutScaling=2^0  OutDataTypeStr=single
  Divide : Product  Inputs=*/  OutDataType=fixdt(1, 16)  OutScaling=2^-10  OutDataTypeStr=Inherit: Inherit via back propagation
  Divide1 : Product  Inputs=**
  Divide2 : Product  Inputs=**
  Divide3 : Product  Inputs=*/
  Divide6 : Product  Inputs=*/  OutDataTypeStr=Inherit: Inherit via back propagation
  Logical Operator : Logic  Operator=NOT  AllPortsSameDT=off  OutDataTypeMode=boolean  LogicDataType=fixdt(0, 8)  OutDataTypeStr=boolean
  Sum of Elements : Sum  Inputs=+  OutDataType=fixdt(1, 16)  OutScaling=2^-10  OutDataTypeStr=Inherit: Inherit via back propagation
  integrator : Defined_Functionality/integrator  SystemSampleTime=-1  Initial_Value=0
  integrator1 : Defined_Functionality/integrator  SystemSampleTime=-1  Initial_Value=0
  integrator2 : Defined_Functionality/integrator  SystemSampleTime=-1  Initial_Value=0
  CORd_c_ChaCRaw : Outport  OutDataType=fixdt(1, 16)  OutScaling=2^0
  CORd_t_ChaTempAvrage : Outport  Port=2  OutDataType=fixdt(1, 16)  OutScaling=2^0
  CORd_i_ChaCurAvrage : Outport  Port=3  OutDataType=fixdt(1, 16)  OutScaling=2^0
  wires:
  Abs/1 -> CORd_c_ChaCRaw/1
  Divide1/1 -> integrator2/1
  integrator2/1 -> Divide6/1
  integrator/1 -> Divide3/2
  Logical Operator/1 -> Average_Current_Calculation/Enable
  CORd_flg_ConstVoltCha/1 -> Logical Operator/1
  Constant6/1 -> Divide6/2
  Divide6/1 -> Abs/1  "CORd_c_ChaCRaw"
  Divide/1 -> CORd_t_ChaTempAvrage/1
  Divide3/1 -> Sum of Elements/1
  Constant/1 -> Divide/2
  Sum of Elements/1 -> Divide/1
  Average_Current_Calculation/1(CORd_i_ChaCurAvrage) -> CORd_i_ChaCurAvrage/1
  [IPTd_i_ShuntCur] -> Average_Current_Calculation/1(IPTd_i_ShuntCur)
  Constant3/1 -> integrator/1
  integrator1/1 -> Divide3/1
  Divide2/1 -> integrator1/1
  Constant2/1 -> Divide2/1
  CORd_t_MdlTemp/1 -> Divide2/2
  Constant1/1 -> Divide1/1
  IPTd_i_ShuntCur/1 -> [IPTd_i_ShuntCur], Divide1/2

== system COR_lib/COR/MainAlgorithm/SOHCalc/SohUpdate/ChaIntSoc ==
  CORd_pct_MdlSoc : Inport
  Enable : EnablePort
  Gain : Gain  ParameterDataType=fixdt(1, 16)  ParameterScaling=2^0  OutDataType=fixdt(1, 16)  OutScaling=2^0
  CORd_pct_ChaInSoc : Outport  OutDataType=fixdt(1, 16)  OutScaling=2^0
  wires:
  Gain/1 -> CORd_pct_ChaInSoc/1
  CORd_pct_MdlSoc/1 -> Gain/1

== system COR_lib/COR/MainAlgorithm/SOHCalc/SohUpdate/ChargingSt ==
  CORd_flg_ChaSt : Inport
  Constant1 : Constant  Value=0  OutDataTypeMode=uint8  OutDataType=fixdt(1, 16)  OutScaling=2^0  OutDataTypeStr=uint8
  Constant2 : Constant  OutDataTypeMode=uint8  OutDataTypeStr=uint8
  Constant3 : Constant  OutDataTypeMode=uint8  OutDataTypeStr=uint8
  Data Store Read : DataStoreRead  DataStoreName=CORd_c_ChaC  SampleTime=-1
  Logical Operator1 : Logic  AllPortsSameDT=off  OutDataTypeMode=boolean  LogicDataType=fixdt(0, 8)  OutDataTypeStr=boolean
  Logical Operator4 : Logic  AllPortsSameDT=off  OutDataTypeMode=boolean  LogicDataType=fixdt(0, 8)  OutDataTypeStr=boolean
  Relational Operator6 : RelationalOperator  Operator=>  LogicOutDataTypeMode=boolean  LogicDataType=fixdt(0, 8)  OutDataTypeStr=boolean
  Relational Operator7 : RelationalOperator  Operator=~=  LogicOutDataTypeMode=boolean  OutDataTypeStr=boolean
  Relational Operator8 : RelationalOperator  Operator===  LogicOutDataTypeMode=boolean  OutDataTypeStr=boolean
  Unit Delay : UnitDelay  SampleTime=-1
  ChargingSt : Outport
  wires:
  Constant1/1 -> Relational Operator6/2
  Data Store Read/1 -> Relational Operator6/1
  Logical Operator1/1 -> ChargingSt/1
  Logical Operator4/1 -> Logical Operator1/1
  CORd_flg_ChaSt/1 -> Relational Operator7/1, Unit Delay/1
  Relational Operator7/1 -> Logical Operator4/1
  Constant2/1 -> Relational Operator7/2
  Constant3/1 -> Relational Operator8/2
  Relational Operator8/1 -> Logical Operator4/2
  Unit Delay/1 -> Relational Operator8/1
  Relational Operator6/1 -> Logical Operator1/2

== system COR_lib/COR/MainAlgorithm/SOHCalc/SohUpdate/ChargingSt1 ==
  CORd_flg_ChaSt : Inport
  Constant2 : Constant  OutDataTypeMode=uint8  OutDataTypeStr=uint8
  Constant3 : Constant  OutDataTypeMode=uint8  OutDataTypeStr=uint8
  Logical Operator4 : Logic  AllPortsSameDT=off  OutDataTypeMode=boolean  LogicDataType=fixdt(0, 8)  OutDataTypeStr=boolean
  Relational Operator7 : RelationalOperator  Operator===  LogicOutDataTypeMode=boolean  OutDataTypeStr=boolean
  Relational Operator8 : RelationalOperator  Operator=~=  LogicOutDataTypeMode=boolean  OutDataTypeStr=boolean
  Unit Delay : UnitDelay  SampleTime=-1
  ChargingSt : Outport
  wires:
  Unit Delay/1 -> Relational Operator8/1
  Relational Operator8/1 -> Logical Operator4/2
  Constant3/1 -> Relational Operator8/2
  Constant2/1 -> Relational Operator7/2
  Relational Operator7/1 -> Logical Operator4/1
  CORd_flg_ChaSt/1 -> Unit Delay/1, Relational Operator7/1
  Logical Operator4/1 -> ChargingSt/1

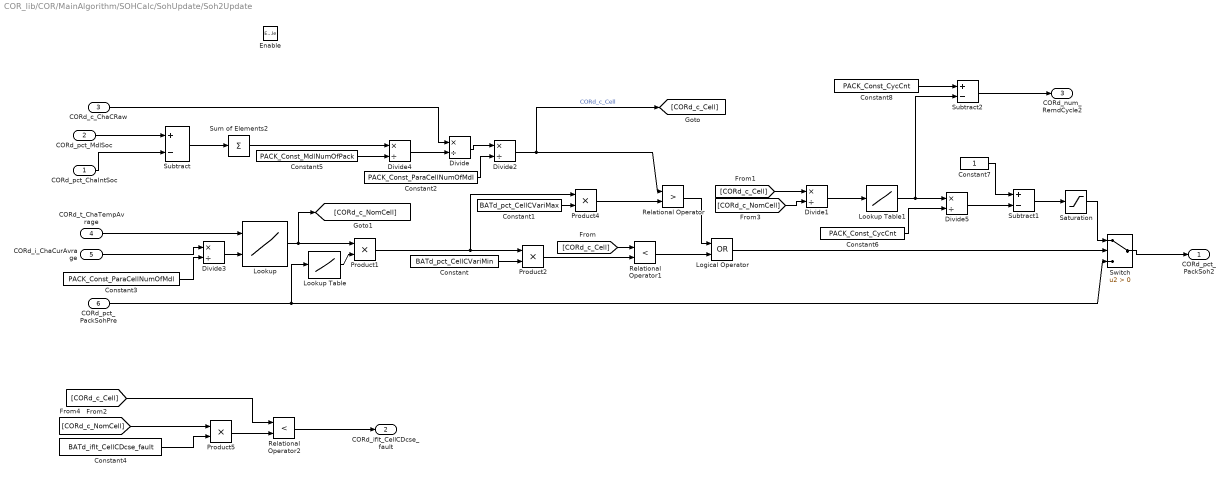
== system COR_lib/COR/MainAlgorithm/SOHCalc/SohUpdate/Soh2Update ==
  CORd_pct_ChaIntSoc : Inport
  CORd_pct_MdlSoc : Inport  Port=2
  CORd_c_ChaCRaw : Inport  Port=3
  CORd_t_ChaTempAvrage : Inport  Port=4
  CORd_i_ChaCurAvrage : Inport  Port=5
  CORd_pct_PackSohPre : Inport  Port=6
  Enable : EnablePort
  Constant : Constant  Value=BATd_pct_CellCVariMin  OutDataType=fixdt(1, 16)  OutScaling=2^0
  Constant1 : Constant  Value=BATd_pct_CellCVariMax  OutDataType=fixdt(1, 16)  OutScaling=2^0
  Constant2 : Constant  Value=PACK_Const_ParaCellNumOfMdl  OutDataTypeMode=single  OutDataType=fixdt(1, 16)  OutScaling=2^0  OutDataTypeStr=single
  Constant3 : Constant  Value=PACK_Const_ParaCellNumOfMdl  OutDataTypeMode=single  OutDataType=fixdt(1, 16)  OutScaling=2^0  OutDataTypeStr=single
  Constant4 : Constant  Value=BATd_iflt_CellCDcse_fault  OutDataTypeMode=single  OutDataType=fixdt(1, 16)  OutScaling=2^0  OutDataTypeStr=single
  Constant5 : Constant  Value=PACK_Const_MdlNumOfPack  OutDataTypeMode=single  OutDataType=fixdt(1, 16)  OutScaling=2^0  OutDataTypeStr=single
  Constant6 : Constant  Value=PACK_Const_CycCnt  OutDataType=fixdt(1, 16)  OutScaling=2^0  OutDataTypeStr=Inherit: Inherit via back propagation
  Constant7 : Constant  OutDataTypeMode=single  OutDataType=fixdt(1, 16)  OutScaling=2^0  OutDataTypeStr=single
  Constant8 : Constant  Value=PACK_Const_CycCnt  OutDataType=fixdt(1, 16)  OutScaling=2^0  OutDataTypeStr=Inherit: Inherit via back propagation
  Divide{,1..5} (6 alike) : Product  Inputs=*/  OutDataType=fixdt(1, 16)  OutScaling=2^-10
  Logical Operator : Logic  Operator=OR  AllPortsSameDT=off  OutDataTypeMode=boolean  LogicDataType=fixdt(0, 8)  OutDataTypeStr=boolean
  Lookup : Lookup2D  RowIndex=BATx_t_CellChaTemp  ColumnIndex=BATy_i_CellChaCur  Table=BATm_c_CellChaC_AH  OutDataTypeMode=single  OutDataType=fixdt(1, 16)  OutScaling=2^0  OutDataTypeStr=single
  Lookup Table : Lookup  InputValues=BATx_pct_PackSoh  Table=BATm_pct_CellCDcseRatio  OutDataType=fixdt(1, 16)  OutScaling=2^0
  Lookup Table1 : Lookup  InputValues=BATx_pct_CellSocRatio  Table=BATm_pct_CellCycle  OutDataType=fixdt(1, 16)  OutScaling=2^0
  Product{1..2,4..5} (4 alike) : Product  OutDataType=fixdt(1, 16)  OutScaling=2^0  RndMeth=Zero
  Relational Operator : RelationalOperator  Operator=>  LogicOutDataTypeMode=boolean  LogicDataType=fixdt(0, 8)  OutDataTypeStr=boolean
  Relational Operator1 : RelationalOperator  Operator=<  LogicOutDataTypeMode=boolean  LogicDataType=fixdt(0, 8)  OutDataTypeStr=boolean
  Relational Operator2 : RelationalOperator  Operator=<  LogicOutDataTypeMode=boolean  LogicDataType=fixdt(0, 8)  OutDataTypeStr=boolean
  Saturation : Saturate  UpperLimit=1  LowerLimit=0  OutDataType=fixdt(1, 16)  OutScaling=2^0
  Subtract : Sum  Inputs=+-  OutDataType=fixdt(1, 16)  OutScaling=2^-10
  Subtract1 : Sum  Inputs=+-  OutDataType=fixdt(1, 16)  OutScaling=2^-10
  Subtract2 : Sum  Inputs=+-  OutDataType=fixdt(1, 16)  OutScaling=2^-10
  Sum of Elements2 : Sum  Inputs=+  OutDataType=fixdt(1, 16)  OutScaling=2^-10
  Switch : Switch  Criteria=u2 > Threshold  OutDataType=fixdt(1, 16)  OutScaling=2^0
  CORd_pct_PackSoh2 : Outport  OutDataType=fixdt(1, 16)  OutScaling=2^0
  CORd_iflt_CellCDcse_fault : Outport  Port=2  OutDataType=fixdt(1, 16)  OutScaling=2^0
  CORd_num_RemdCycle2 : Outport  Port=3  OutDataType=fixdt(1, 16)  OutScaling=2^0
  wires:
  Divide4/1 -> Divide/2
  Subtract/1 -> Sum of Elements2/1
  Constant5/1 -> Divide4/2
  Sum of Elements2/1 -> Divide4/1
  Divide2/1 -> Relational Operator/1, [CORd_c_Cell]  "CORd_c_Cell"
  Saturation/1 -> Switch/1
  Switch/1 -> CORd_pct_PackSoh2/1
  Constant4/1 -> Product5/2
  Relational Operator2/1 -> CORd_iflt_CellCDcse_fault/1
  [CORd_c_Cell] -> Relational Operator2/1
  [CORd_c_NomCell] -> Product5/1
  Product5/1 -> Relational Operator2/2
  Constant3/1 -> Divide3/2
  Divide3/1 -> Lookup/2
  CORd_i_ChaCurAvrage/1 -> Divide3/1
  Constant2/1 -> Divide2/2
  Divide/1 -> Divide2/1
  Divide1/1 -> Lookup Table1/1
  Lookup Table/1 -> Product1/2
  [CORd_c_NomCell] -> Divide1/2
  [CORd_c_Cell] -> Divide1/1
  Logical Operator/1 -> Switch/2
  Relational Operator1/1 -> Logical Operator/2
  Relational Operator/1 -> Logical Operator/1
  Product2/1 -> Relational Operator1/2
  [CORd_c_Cell] -> Relational Operator1/1
  Product4/1 -> Relational Operator/2
  Constant1/1 -> Product4/2
  Constant/1 -> Product2/2
  Product1/1 -> Product4/1, Product2/1
  CORd_pct_PackSohPre/1 -> Lookup Table/1, Switch/3
  Lookup/1 -> [CORd_c_NomCell], Product1/1
  CORd_t_ChaTempAvrage/1 -> Lookup/1
  CORd_c_ChaCRaw/1 -> Divide/1
  CORd_pct_ChaIntSoc/1 -> Subtract/2
  CORd_pct_MdlSoc/1 -> Subtract/1
  Lookup Table1/1 -> Divide5/1, Subtract2/2
  Constant6/1 -> Divide5/2
  Subtract1/1 -> Saturation/1
  Divide5/1 -> Subtract1/2
  Constant7/1 -> Subtract1/1
  Constant8/1 -> Subtract2/1
  Subtract2/1 -> CORd_num_RemdCycle2/1

== system COR_lib/COR/MainAlgorithm/SOHCalc/SohUpdate/ChaCapacityCal/Average_Current_Calculation ==
  IPTd_i_ShuntCur : Inport
  Enable : EnablePort
  Constant4 : Constant  Value=BMS_Const_TickTm_s  OutDataTypeMode=single  OutDataType=fixdt(1, 16)  OutScaling=2^0  OutDataTypeStr=single
  Constant5 : Constant  Value=BMS_Const_TickTm_s  OutDataTypeMode=single  OutDataType=fixdt(1, 16)  OutScaling=2^0  OutDataTypeStr=single
  Divide4 : Product  Inputs=**
  Divide5 : Product  Inputs=*/
  integrator : Defined_Functionality/integrator  SystemSampleTime=-1  Initial_Value=0
  integrator1 : Defined_Functionality/integrator  SystemSampleTime=-1  Initial_Value=0
  CORd_i_ChaCurAvrage : Outport
  wires:
  Divide4/1 -> integrator1/1
  integrator1/1 -> Divide5/1
  integrator/1 -> Divide5/2
  IPTd_i_ShuntCur/1 -> Divide4/2
  Divide5/1 -> CORd_i_ChaCurAvrage/1
  Constant5/1 -> integrator/1
  Constant4/1 -> Divide4/1
